simulink model "fxpdemo_parallel_form"  (Simulink 5.0)
settings: Solver=FixedStepDiscrete  SolverMode=SingleTasking  StartTime=0.0  StopTime=200  FixedStep=1  RelTol=1e-3
libraries: fixpt_lib_4 x2
settings Model: CovMetricSettings=d  MinMaxOverflowLogging=MinMaxAndOverflow  Creator=andyb  LastModifiedBy=andyb  ExtModeTrigMode=oneshot  ExtModeArmWhenConnect=off  ExtModeAutoUpdateStatusClock=off  LimitDataPoints=off  IntegerOverflowMsg=none  ParameterDowncastMsg=warning  ParameterOverflowMsg=warning  ParameterPrecisionLossMsg=none  RTWInlineParameters=on  RTWOptions="-aEnforceIntegerDowncast=1 -aExtMode=0 -aExtModeTesting=0 -aFoldNonRolledExpr=1 -aForceParamTrailComments=0 -aGenerateComments=1 -aGenerateReport=1 -aIgnoreCustomStorageClasses=1 -aIncDataTypeInIds=0 -aIncHierarchyInIds=0 -aInlineInvariantSignals=1 -aInlinedPrmAccess=\"Literals\" -aLocalBlockOutputs=1 -aLogVarNameModifier=\"rt_\" -aMaxRTWIdLen=31 -aPrefixModelToSubsysFcnNames=1 -aRTWVerbose=1 -aRollThreshold=5 -aShowEliminatedStatements=1"

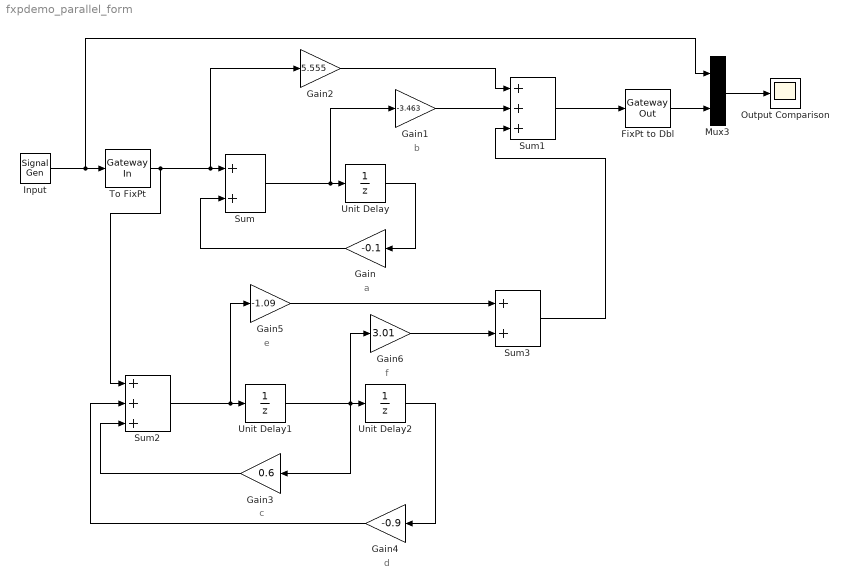
== system fxpdemo_parallel_form ==
  note: b
  note: a
  note: e
  note: f
  note: c
  note: d
  FixPt to Dbl : fixpt_lib_4/Data Type/Gateway Out  OutRealWorld=Real World Value  OutBuiltInType=double  DoSatur=off
  Gain : Gain  Orientation=left  Gain=-0.1  ShowAdditionalParam=on  ParameterDataTypeMode=Specify via dialog  ParameterDataType=sfix( 16 )  ParameterScalingMode=Best Precision: Column-wise  ParameterScaling=2^-18  OutDataTypeMode=Specify via dialog  OutScaling=2^-10
  Gain1 : Gain  Gain=-3.463  ShowAdditionalParam=on  ParameterDataTypeMode=Specify via dialog  ParameterDataType=sfix( 16 )  ParameterScalingMode=Best Precision: Column-wise  ParameterScaling=2^-13  OutDataTypeMode=Specify via dialog  OutScaling=2^-10
  Gain2 : Gain  Gain=5.555  ShowAdditionalParam=on  ParameterDataTypeMode=Specify via dialog  ParameterDataType=sfix( 16 )  ParameterScalingMode=Best Precision: Column-wise  ParameterScaling=2^-12  OutDataTypeMode=Specify via dialog  OutScaling=2^-10
  Gain3 : Gain  Orientation=left  Gain=0.6  ShowAdditionalParam=on  ParameterDataTypeMode=Specify via dialog  ParameterDataType=sfix( 16 )  ParameterScalingMode=Best Precision: Column-wise  ParameterScaling=2^-15  OutDataTypeMode=Specify via dialog  OutScaling=2^-10
  Gain4 : Gain  Orientation=left  Gain=-0.9  ShowAdditionalParam=on  ParameterDataTypeMode=Specify via dialog  ParameterDataType=sfix( 16 )  ParameterScalingMode=Best Precision: Column-wise  ParameterScaling=2^-15  OutDataTypeMode=Specify via dialog  OutScaling=2^-10
  Gain5 : Gain  Gain=-1.09  ShowAdditionalParam=on  ParameterDataTypeMode=Specify via dialog  ParameterDataType=sfix( 16 )  ParameterScalingMode=Best Precision: Column-wise  ParameterScaling=2^-14  OutDataTypeMode=Specify via dialog  OutScaling=2^-10
  Gain6 : Gain  Gain=3.01  ShowAdditionalParam=on  ParameterDataTypeMode=Specify via dialog  ParameterDataType=sfix( 16 )  ParameterScalingMode=Best Precision: Column-wise  ParameterScaling=2^-13  OutDataTypeMode=Specify via dialog  OutScaling=2^-10
  Input : SignalGenerator  WaveForm=square  Frequency=0.005
  Mux3 : Mux  Inputs=2
  Output Comparison : Scope
      settings: TickLabels=on  TimeRange=200  YMin=-8  YMax=10  SaveName=OutputComparison
  Sum : Sum  ShowAdditionalParam=on  OutDataTypeMode=Specify via dialog  OutScaling=2^-10
  Sum1 : Sum  Inputs=+++  ShowAdditionalParam=on  OutDataTypeMode=Specify via dialog  OutScaling=2^-10
  Sum2 : Sum  Inputs=+++  ShowAdditionalParam=on  OutDataTypeMode=Specify via dialog  OutScaling=2^-10
  Sum3 : Sum  ShowAdditionalParam=on  OutDataTypeMode=Specify via dialog  OutScaling=2^-10
  To FixPt : fixpt_lib_4/Data Type/Gateway In  InRealWorld=Real World Value  OutputDataTypeScalingMode=Specify via dialog  OutDataType=sfix(16)  OutScaling=2^-10  DoSatur=off
  Unit Delay : UnitDelay  X0=0.0  SampleTime=1.0
  Unit Delay1 : UnitDelay  X0=0.0  SampleTime=1.0
  Unit Delay2 : UnitDelay  X0=0.0  SampleTime=1.0
  wires:
  Input/1 -> To FixPt/1, Mux3/1
  Gain/1 -> Sum/2
  Sum/1 -> Unit Delay/1, Gain1/1
  Gain1/1 -> Sum1/2
  Gain2/1 -> Sum1/1
  Sum1/1 -> FixPt to Dbl/1
  Mux3/1 -> Output Comparison/1
  FixPt to Dbl/1 -> Mux3/2
  To FixPt/1 -> Sum/1, Gain2/1, Sum2/1
  Unit Delay/1 -> Gain/1
  Gain3/1 -> Sum2/3
  Sum2/1 -> Unit Delay1/1, Gain5/1
  Unit Delay1/1 -> Unit Delay2/1, Gain3/1, Gain6/1
  Gain4/1 -> Sum2/2
  Sum3/1 -> Sum1/3
  Gain6/1 -> Sum3/2
  Gain5/1 -> Sum3/1
  Unit Delay2/1 -> Gain4/1
